simulink model "WiperSystem"  (R2022b)
settings: Solver=FixedStepDiscrete  StartTime=0.0  StopTime=20.0  FixedStep=0.01  RelTol=1e-3
undefined symbols (not defined in the file): sigbuilder_block
libraries: simulink x1
settings Model: Creator=Mohamed Youness  LastModifiedBy=Mohamed Youness

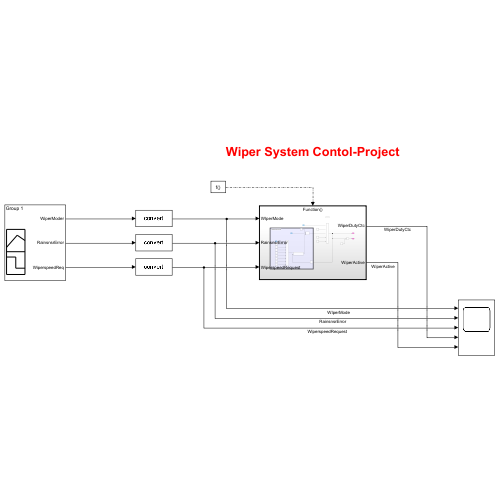
[thumbnail: Simulink's stored preview of the top-level diagram]
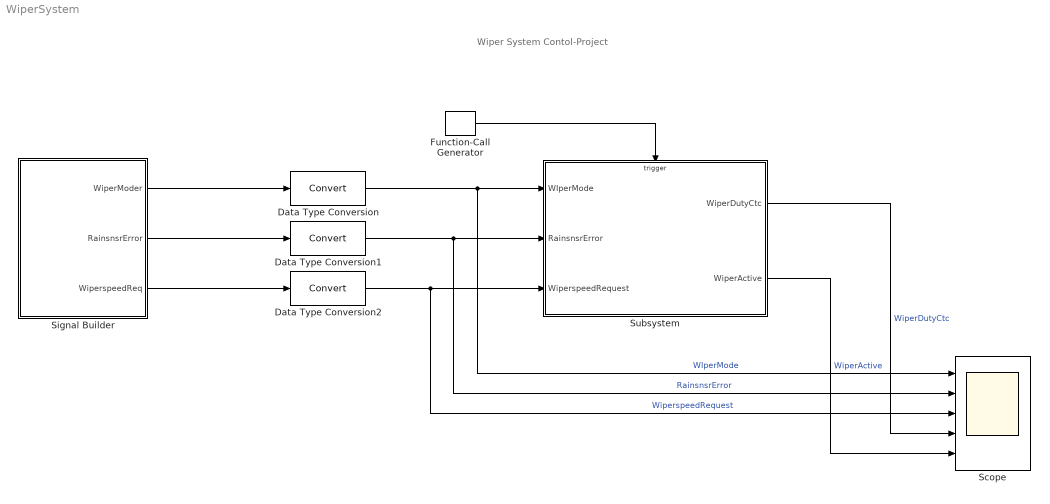
== system WiperSystem ==
  note: Wiper System Contol-Project
  Data Type Conversion : DataTypeConversion  SaturateOnIntegerOverflow=off  RndMeth=Floor
  Data Type Conversion1 : DataTypeConversion  SaturateOnIntegerOverflow=off  RndMeth=Floor
  Data Type Conversion2 : DataTypeConversion  SaturateOnIntegerOverflow=off  RndMeth=Floor
  Function-Call Generator : simulink/Ports & Subsystems/Function-Call Generator  sample_time=10e-3  numberOfIterations=1  DisallowWideOutput=off
  Scope : Scope  NumInputPorts=5
  Signal Builder : Subsystem  Tag=STV Subsys  LoadFcn=sigbuilder_block('load');  StartFcn=sigbuilder_block('start');  StopFcn=sigbuilder_block('stop');  ClipboardFcn=sigbuilder_block('clipboard');  mask(Sigbuilder block){tuvar=[0:10]}
      mask help: Simulink:masks:SigbuilderBlock_MD
      mask init:
      | if ~strcmp(get_param(bdroot(gcbh),'SimulationStatus'),'stopped') tuvar = sigbuilder_block('maskInit'); end
      settings: CopyFcn=sigbuilder_block('copy');  DeleteFcn=sigbuilder_block('delete');  ModelCloseFcn=sigbuilder_block('modelClose');  PreSaveFcn=sigbuilder_block('preSave');  PauseFcn=sigbuilder_block('pause');  ContinueFcn=sigbuilder_block('continue');  NameChangeFcn=sigbuilder_block('namechange');  OpenFcn=sigbuilder_block('open',[0.6 36.6 574.8 549.6 ]);  CloseFcn=sigbuilder_block('close');
      mask Display: plot(0, 0, 100, 100,[2, 2, 32, 32, 2], [68, 8, 8, 68, 68],[32, 2], [38, 38], [32, 19, 2],[53, 60, 44], [32, 17, 17, 2],[16, 16, 31, 31]);txt = getActiveGroup(gcbh);text(2, 100, txt,'verticalAlignment', 'top');
  Subsystem : Subsystem
  wires:
  Data Type Conversion/1 -> Scope/1, Subsystem/1(WIperMode)  "WIperMode"
  Data Type Conversion1/1 -> Scope/2, Subsystem/2(RainsnsrError)  "RainsnsrError"
  Data Type Conversion2/1 -> Scope/3, Subsystem/3(WiperspeedRequest)  "WiperspeedRequest"
  Subsystem/1(WiperDutyCtc) -> Scope/4  "WiperDutyCtc"
  Subsystem/2(WiperActive) -> Scope/5  "WiperActive"
  Function-Call Generator/1 -> Subsystem/Trigger
  Signal Builder/1(WiperModer) -> Data Type Conversion/1
  Signal Builder/2(RainsnsrError) -> Data Type Conversion1/1
  Signal Builder/3(WiperspeedReq) -> Data Type Conversion2/1

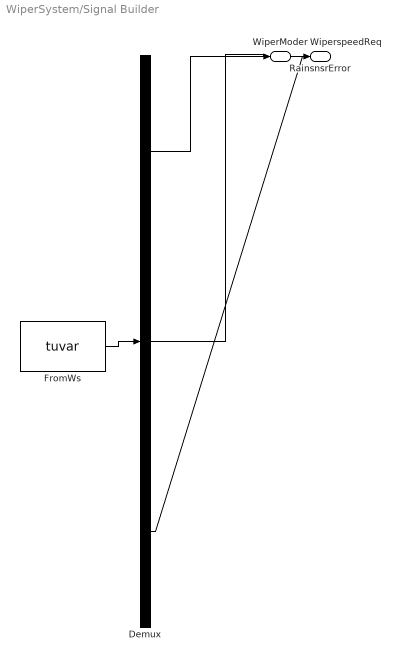
== system WiperSystem/Signal Builder ==
  Demux : Demux  Tag=STV Demux  Outputs=3
      settings: DisplayOption=none
  FromWs : FromWorkspace  Tag=STV FromWs  VariableName=tuvar
      SigBuilderData=|
      | common.afterFinalStr = 'Extrapolate'
      | common.sampleTime = 0
      | dataSet.timeRange = [0 20]
      | dataSet.name = 'Group 1'
      | sbobj.Groups.Name = 'Group 1'
      | sbobj.Groups.Signals(1).Name = 'WiperModer'
      | sbobj.Groups.Signals(1).XData = [0 2 2 4 4 6 6 7 8 9 10 11 12 13 14 15 20]
      | sbobj.Groups.Signals(1).YData = [0 0 2 2 3 3 1 1 1 1 1 1 1 1 1 1 1]
      | sbobj.Groups.Signals(2).Name = 'RainsnsrError'
      | sbobj.Groups.Signals(2).XData = [0 14 15 16 20]
      | sbobj.Groups.Signals(2).YData = [0 0 1 0 0]
      | sbobj.Groups.Signals(3).Name = 'WiperspeedReq'
      | sbobj.Groups.Signals(3).XData = [0 7 14 20]
      | sbobj.Groups.Signals(3).YData = [0 0 7 7]
      | sbobj.Groups.TimeRange = [0 20]
  WiperModer : Outport  Tag=STV Outport
  RainsnsrError : Outport  Tag=STV Outport  Port=2
  WiperspeedReq : Outport  Tag=STV Outport  Port=3
  wires:
  Demux/1 -> WiperModer/1
  FromWs/1 -> Demux/1
  Demux/2 -> RainsnsrError/1
  Demux/3 -> WiperspeedReq/1

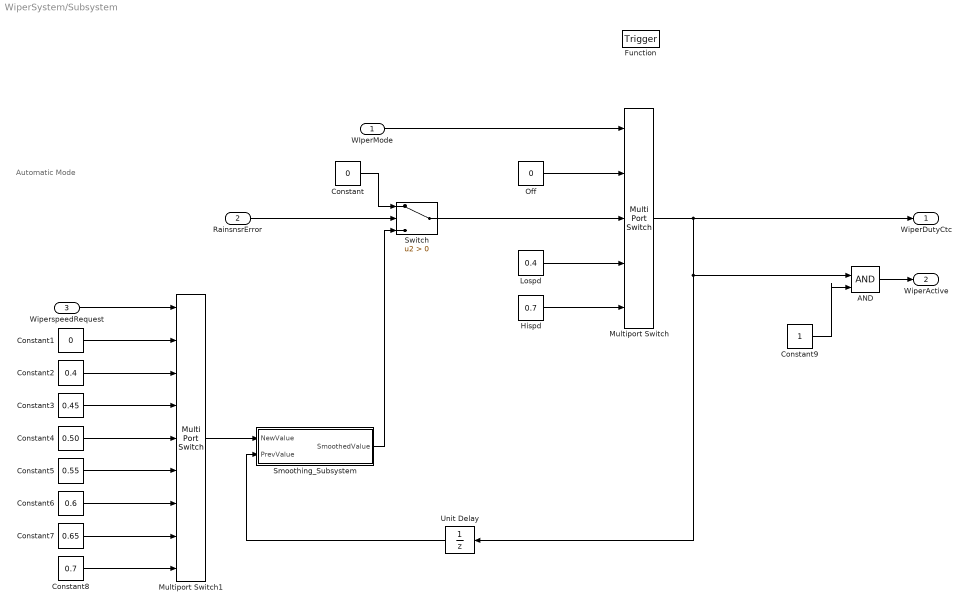
== system WiperSystem/Subsystem ==
  note: Automatic Mode
  WIperMode : Inport  OutDataTypeStr=uint8
  RainsnsrError : Inport  Port=2  OutDataTypeStr=boolean
  WiperspeedRequest : Inport  Port=3  OutDataTypeStr=uint8
  Function : TriggerPort  TriggerType=function-call  VariantControl=(inherit)  PortDimensions=1
  AND : Logic  IconShape=distinctive  AllPortsSameDT=off  OutDataTypeStr=boolean
  Constant : Constant  Value=0
  Constant1 : Constant  Value=0
  Constant2 : Constant  Value=0.4
  Constant3 : Constant  Value=0.45
  Constant4 : Constant  Value=0.50
  Constant5 : Constant  Value=0.55
  Constant6 : Constant  Value=0.6
  Constant7 : Constant  Value=0.65
  Constant8 : Constant  Value=0.7
  Constant9 : Constant
  Hispd : Constant  Value=0.7
  Lospd : Constant  Value=0.4
  Multiport Switch : MultiPortSwitch  DataPortOrder=Zero-based contiguous  Inputs=4  zeroidx=on  OutDataTypeStr=single  SaturateOnIntegerOverflow=off  InputSameDT=off
  Multiport Switch1 : MultiPortSwitch  DataPortOrder=Zero-based contiguous  Inputs=8  zeroidx=on  SaturateOnIntegerOverflow=off  InputSameDT=off
  Off : Constant  Value=0
  Smoothing_Subsystem : Subsystem
  Switch : Switch  Criteria=u2 > Threshold  SaturateOnIntegerOverflow=off  InputSameDT=off
  Unit Delay : UnitDelay  SampleTime=-1  HasFrameUpgradeWarning=on
  WiperDutyCtc : Outport  OutDataTypeStr=single
  WiperActive : Outport  Port=2  OutDataTypeStr=boolean
  wires:
  Lospd/1 -> Multiport Switch/4
  WIperMode/1 -> Multiport Switch/1
  Hispd/1 -> Multiport Switch/5
  Constant/1 -> Switch/1
  Constant5/1 -> Multiport Switch1/6
  Constant2/1 -> Multiport Switch1/3
  Multiport Switch/1 -> WiperDutyCtc/1, Unit Delay/1, AND/1
  Off/1 -> Multiport Switch/2
  RainsnsrError/1 -> Switch/2
  AND/1 -> WiperActive/1
  WiperspeedRequest/1 -> Multiport Switch1/1
  Constant1/1 -> Multiport Switch1/2
  Multiport Switch1/1 -> Smoothing_Subsystem/1(NewValue)
  Switch/1 -> Multiport Switch/3
  Smoothing_Subsystem/1(SmoothedValue) -> Switch/3
  Constant9/1 -> AND/2
  Constant3/1 -> Multiport Switch1/4
  Constant4/1 -> Multiport Switch1/5
  Constant7/1 -> Multiport Switch1/8
  Constant6/1 -> Multiport Switch1/7
  Constant8/1 -> Multiport Switch1/9
  Unit Delay/1 -> Smoothing_Subsystem/2(PrevValue)

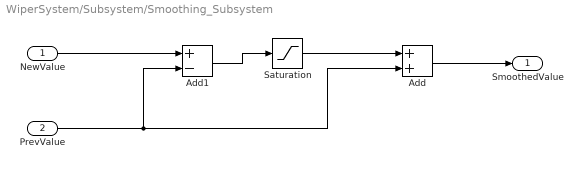
== system WiperSystem/Subsystem/Smoothing_Subsystem ==
  NewValue : Inport
  PrevValue : Inport  Port=2
  Add : Sum
  Add1 : Sum  Inputs=+-
  Saturation : Saturate  UpperLimit=0.005  LowerLimit=-0.005
  SmoothedValue : Outport
  wires:
  NewValue/1 -> Add1/1
  PrevValue/1 -> Add1/2, Add/2
  Add1/1 -> Saturation/1
  Saturation/1 -> Add/1
  Add/1 -> SmoothedValue/1
